simulink model "TestodestoTogether"  (R2025b)
settings: Solver=VariableStepAuto  StartTime=0.0  StopTime=800  RelTol=1e-3
values from neighbouring files (symbols this model uses):
  A_sym_calc = sym(A_num)    [calculate_system.m]
  B_sym_calc = sym(B_num)    [calculate_system.m]
  C_sym_calc = sym(C_num)    [calculate_system.m]
settings Model: Creator=fabim  LastModifiedBy=fabim

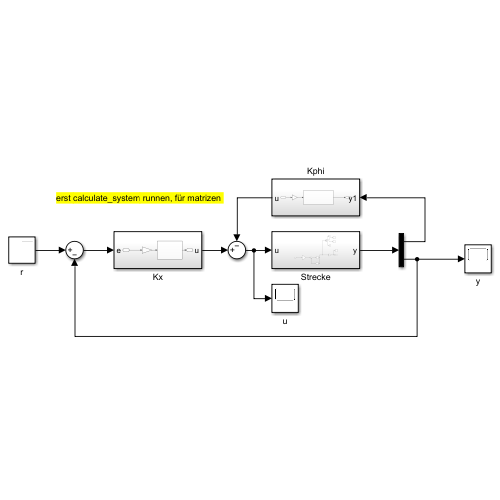
[thumbnail: Simulink's stored preview of the top-level diagram]
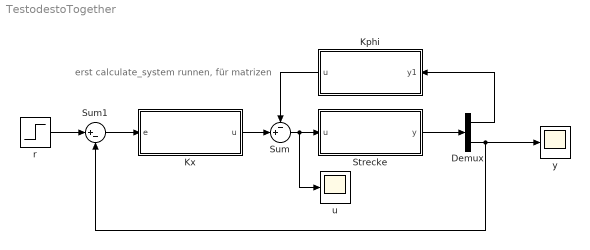
== system TestodestoTogether ==
  note: erst calculate_system runnen, für matrizen
  Demux : Demux  Outputs=2
  Kphi : Subsystem
  Kx : Subsystem
  Strecke : Subsystem
  Sum : Sum  Inputs=-+|
  Sum1 : Sum  Inputs=|+-
  r : Step  Time=400  SampleTime=0
  u : Scope
      settings: ActiveDisplayYMinimum=-1  ActiveDisplayYMaximum=1  DataLoggingVariableName=ScopeData4
  y : Scope
      settings: ActiveDisplayYMinimum=-0.3038313780972467  ActiveDisplayYMaximum=1.9823492541316843  DataLoggingVariableName=ScopeData3
  wires:
  Strecke/1(y) -> Demux/1
  Demux/2 -> Sum1/2, y/1
  Sum/1 -> u/1, Strecke/1(u)
  Sum1/1 -> Kx/1(e)
  Demux/1 -> Kphi/1(y1)
  Kphi/1(u) -> Sum/1
  Kx/1(u) -> Sum/2
  r/1 -> Sum1/1

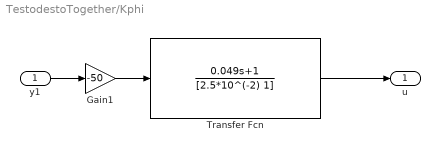
== system TestodestoTogether/Kphi ==
  y1 : Inport
  Gain1 : Gain  Gain=-50
  Transfer Fcn : TransferFcn  Numerator=[0.049 1]  Denominator=[2.5*10^(-2) 1]
  u : Outport
  wires:
  Gain1/1 -> Transfer Fcn/1
  Transfer Fcn/1 -> u/1
  y1/1 -> Gain1/1

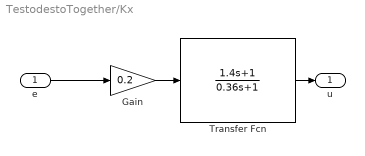
== system TestodestoTogether/Kx ==
  e : Inport
  Gain : Gain  Gain=0.2
  Transfer Fcn : TransferFcn  Numerator=[1.4 1]  Denominator=[0.36 1]
  u : Outport
  wires:
  Gain/1 -> Transfer Fcn/1
  Transfer Fcn/1 -> u/1
  e/1 -> Gain/1

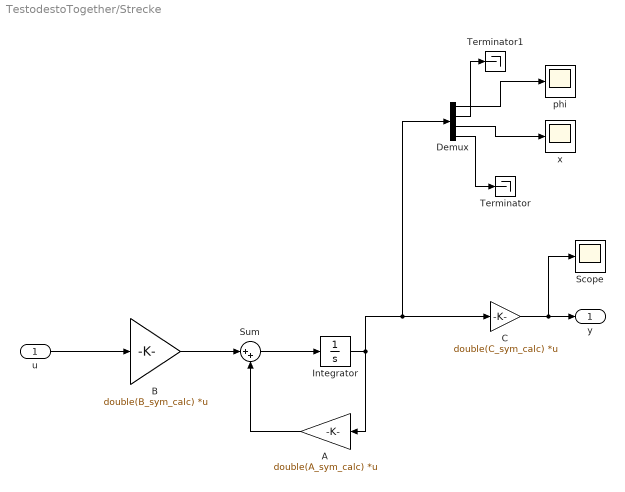
== system TestodestoTogether/Strecke ==
  u : Inport
  A : Gain  Gain=double(A_sym_calc)  Multiplication=Matrix(K*u)
  B : Gain  Gain=double(B_sym_calc)  Multiplication=Matrix(K*u)
  C : Gain  Gain=double(C_sym_calc)  Multiplication=Matrix(K*u)
  Demux : Demux
  Integrator : Integrator  InitialCondition=[0.1;0;0;0]
  Scope : Scope
      settings: ActiveDisplayYMinimum=-0.096422387436448709  ActiveDisplayYMaximum=0.0692669900128686
  Sum : Sum  Inputs=|++
  Terminator : Terminator
  Terminator1 : Terminator
  phi : Scope
      settings: ActiveDisplayYMinimum=-0.060170355003542994  ActiveDisplayYMaximum=0.072892092984425186
  x : Scope
      settings: ActiveDisplayYMinimum=-0.12609102571146941  ActiveDisplayYMaximum=0.1540604441377027  DataLoggingVariableName=ScopeData2
  y : Outport
  wires:
  Sum/1 -> Integrator/1
  A/1 -> Sum/2
  B/1 -> Sum/1
  u/1 -> B/1
  Integrator/1 -> A/1, Demux/1, C/1
  C/1 -> Scope/1, y/1
  Demux/1 -> phi/1
  Demux/3 -> x/1
  Demux/4 -> Terminator/1
  Demux/2 -> Terminator1/1
